simulink model "Sample594"  (R2021b)
settings: Solver=VariableStepAuto  StartTime=0.0  StopTime=10.0  RelTol=1e-3
undefined symbols (not defined in the file): DiscIntNeverNeededParam, magnitude, Newton, Raphson
libraries: simulink x402, pid_lib x98
(part 11 of 14)

== system Sample594/cfblk7/cfblk10/cfblk9/cfblk8 ==
  cfblk1 : Inport
  cfblk6 : Inport  Port=2
  cfblk7 : Inport  Port=3
  cfblk8 : Inport  Port=4
  cfblk3 : simulink/Discrete/Difference  ICPrevInput=0.0  OutMin=[]  OutMax=[]  OutDataTypeStr=Inherit: Inherit via back propagation  OutDataType=fixdt(1, 16)  OutScaling=2^-10  DoSatur=off
  cfblk4 : Sqrt  Operator=rSqrt  AlgorithmType=Newton-Raphson  SaturateOnIntegerOverflow=on
  cfblk5 : Squeeze
  cfblk2 : Outport
  wires:
  cfblk1/1 -> cfblk4/1
  cfblk3/1 -> cfblk2/1
  cfblk6/1 -> cfblk5/1
  cfblk8/1 -> cfblk3/1

== system Sample594/cfblk7/cfblk10/cfblk9/cfblk9 ==
  cfblk1 : Inport
  cfblk11 : Inport  Port=2
  cfblk12 : Inport  Port=3
  cfblk13 : Inport  Port=4
  cfblk14 : Inport  Port=5
  cfblk15 : Inport  Port=6
  cfblk16 : Inport  Port=7
  cfblk10 : simulink/Math Operations/MinMax Running Resettable  Function=min  vinit=0.0
  cfblk18 : Delay  SampleTime=1
  cfblk3 : simulink/Discrete/Tapped Delay  vinit=0.0  samptime=-1  NumDelays=1  DelayOrder=Oldest  includeCurrent=off
  cfblk4 : pid_lib/PID Controller (2DOF)  Controller=PID  Form=Parallel  TimeDomain=Discrete-time  UseExternalTs=off  SampleTime=1  IntegratorMethod=Forward Euler  FilterMethod=Forward Euler  ControllerParametersSource=internal  P=1  I=1  D=0  UseFilter=on  N=100  b=1  c=1  TunerSelectOption=Transfer Function Based (PID Tuner App)  InitialConditionSource=internal  InitialConditionForIntegrator=0  InitialConditionForFilter=0  DifferentiatorICPrevScaledInput=0  ExternalReset=none  TrackingMode=off  Kt=1  LimitOutput=off  SatLimitsSource=internal  UpperSaturationLimit=inf  LowerSaturationLimit=-inf  LinearizeAsGain=off  AntiWindupMode=none  Kb=1  POutMin=[]  POutMax=[]  IOutMin=[]  IOutMax=[]  DOutMin=[]  DOutMax=[]  NOutMin=[]  NOutMax=[]  bOutMin=[]  bOutMax=[]  cOutMin=[]  cOutMax=[]  SumOutMin=[]  SumOutMax=[]  SaturationOutMin=[]  SaturationOutMax=[]  PParamMin=[]  PParamMax=[]  IParamMin=[]  IParamMax=[]  DParamMin=[]  DParamMax=[]  NParamMin=[]  NParamMax=[]  bParamMin=[]  bParamMax=[]  cParamMin=[]  cParamMax=[]  KbParamMin=[]  KbParamMax=[]  KtParamMin=[]  KtParamMax=[]  KbOutMin=[]  KbOutMax=[]  KtOutMin=[]  KtOutMax=[]  IntegratorOutMin=[]  IntegratorOutMax=[]  FilterOutMin=[]  FilterOutMax=[]  SumI1OutMin=[]  SumI1OutMax=[]  SumI2OutMin=[]  SumI2OutMax=[]  SumI3OutMin=[]  SumI3OutMax=[]  SumI4OutMin=[]  SumI4OutMax=[]  SumDOutMin=[]  SumDOutMax=[]  Sum1OutMin=[]  Sum1OutMax=[]  Sum2OutMin=[]  Sum2OutMax=[]  Sum3OutMin=[]  Sum3OutMax=[]  DifferentiatorOutMin=[]  DifferentiatorOutMax=[]  FilterDiffOutCoefMin=[]  FilterDiffOutCoefMax=[]  ReciprocalOutMin=[]  ReciprocalOutMax=[]  SumDenOutMin=[]  SumDenOutMax=[]  SumNumOutMin=[]  SumNumOutMax=[]  DivideOutMin=[]  DivideOutMax=[]  UdiffTsProdOutMin=[]  UdiffTsProdOutMax=[]  NTsProdOutMin=[]  NTsProdOutMax=[]  UintegralTsProdOutMin=[]  UintegralTsProdOutMax=[]  UngainTsProdOutMin=[]  UngainTsProdOutMax=[]  IntegratorContinuousStateAttributes=''  IntegratorStateMustResolveToSignalObject=off  IntegratorRTWStateStorageClass=Auto  FilterContinuousStateAttributes=''  FilterStateMustResolveToSignalObject=off  FilterRTWStateStorageClass=Auto  ParallelPVariant=InternalParameters  IdealPVariant=Disabled  IVariant=InternalParameters  DVariant=InternalParameters  bVariant=InternalParameters  cVariant=InternalParameters  IntegratorVariant=Discrete  SatVariant=Disabled  AWVariant=Passthrough  PCopyVariant=Disabled  TRVariant=Disabled  FdbkBlocksVariant=Forward  IdealPFdbkVariant=Disabled  SatFdbkVariant=Disabled  DerivativeFilterVariant=ForwardEulerFilter  NVariant=InternalParameters  NCopyVariant=Disabled  FilterICVariant=InternalICsFilter  IntegratorICVariant=InternalICs  ExternalResetVariant=Disabled  TRSumVariant=Passthrough  SumFdbkVariant=Disabled  SumVariant=Sum_PID  TsampFilterVariant=InternalTs  TsampNgainVariant=Passthrough  TsampIntegralVariant=Passthrough  ExternalSaturationOutDataTypeStr=Inherit: Same as second input
      settings: SourceProductBaseCode=SL
  cfblk5 : DotProduct  InputSameDT=on  OutDataTypeStr=Inherit: Inherit via internal rule
  cfblk6 : ComplexToMagnitudeAngle
  cfblk7 : Product  Inputs=**
  cfblk8 : Assignment  DiagnosticForDimensions=Warning  IndexOptions=Index vector (dialog)  Indices=1  OutputSizes=1
  cfblk9 : Bias  Bias=[987332324.215911]
  cfblk2 : Outport
  cfblk17 : Outport  Port=2
  wires:
  cfblk3/1 -> cfblk8/1
  cfblk15/1 -> cfblk9/1
  cfblk1/1 -> cfblk4/1
  cfblk12/1 -> cfblk17/1
  cfblk11/1 -> cfblk3/1
  cfblk14/1 -> cfblk6/1
  cfblk9/1 -> cfblk10/1
  cfblk16/1 -> cfblk7/1
  cfblk8/1 -> cfblk10/2
  cfblk5/1 -> cfblk2/1
  cfblk4/1 -> cfblk7/2
  cfblk13/1 -> cfblk5/1
  cfblk7/1 -> cfblk5/2
  cfblk6/1 -> cfblk4/2
  cfblk10/1 -> cfblk18/1
  cfblk18/1 -> cfblk8/2

== system Sample594/cfblk7/cfblk11/cfblk11/cfblk8 ==
  cfblk1 : Inport
  cfblk7 : Inport  Port=2
  cfblk3 : UnaryMinus
  cfblk4 : Sqrt  Operator=rSqrt  AlgorithmType=Newton-Raphson  SaturateOnIntegerOverflow=on
  cfblk5 : Sqrt  Operator=rSqrt  AlgorithmType=Newton-Raphson  SaturateOnIntegerOverflow=on
  cfblk6 : Constant  Value=[773406502.587289]  SampleTime=1
  cfblk2 : Outport
  cfblk8 : Outport  Port=2
  cfblk9 : Outport  Port=3
  wires:
  cfblk6/1 -> cfblk8/1
  cfblk3/1 -> cfblk4/1
  cfblk5/1 -> cfblk2/1
  cfblk1/1 -> cfblk3/1
  cfblk4/1 -> cfblk5/1
  cfblk7/1 -> cfblk9/1

== system Sample594/cfblk7/cfblk11/cfblk9/cfblk8 ==
  cfblk1 : Inport
  cfblk8 : Inport  Port=2
  cfblk9 : Inport  Port=3
  cfblk10 : Delay  SampleTime=1
  cfblk3 : simulink/Discrete/Transfer Fcn Lead or Lag  PoleZ=0.95  ZeroZ=0.75  ICPrevOutput=0.0  ICPrevInput=0.0  DoSatur=off
      settings: SourceProductBaseCode=SL
  cfblk4 : Delay  SampleTime=1
  cfblk5 : Squeeze
  cfblk6 : Sum  Inputs=|++
  cfblk7 : Signum
  cfblk2 : Outport
  wires:
  cfblk6/1 -> cfblk3/1
  cfblk8/1 -> cfblk2/1
  cfblk4/1 -> cfblk7/1
  cfblk3/1 -> cfblk5/1
  cfblk9/1 -> cfblk4/1
  cfblk1/1 -> cfblk6/2
  cfblk5/1 -> cfblk10/1
  cfblk10/1 -> cfblk6/1

== system Sample594/cfblk7/cfblk12/cfblk6/cfblk11 ==
  cfblk1 : Inport
  cfblk10 : Inport  Port=2
  cfblk11 : Inport  Port=3
  cfblk3 : Delay  ShowEnablePort=on  SampleTime=1
      settings: InputPortMap=u0,e6
  cfblk4 : ComplexToMagnitudeAngle
  cfblk5 : Polyval  Coefs=[ +2.081618890e-019, -1.441693666e-014, +4.719686976e-010, -8.536869453e-006, +1.621573104e-001, -8.087801117e+001 ]
  cfblk6 : UnaryMinus
  cfblk7 : Gain  Gain=[975284197.068087]
  cfblk8 : Gain  Gain=[457208272.318980]
  cfblk9 : Constant  Value=[771388824.910894]  SampleTime=1
  cfblk2 : Outport
  cfblk12 : Outport  Port=2
  wires:
  cfblk8/1 -> cfblk3/1
  cfblk9/1 -> cfblk5/1
  cfblk11/1 -> cfblk3/2
  cfblk10/1 -> cfblk8/1
  cfblk4/1 -> cfblk6/1
  cfblk1/1 -> cfblk7/1
  cfblk5/1 -> cfblk12/1
  cfblk6/1 -> cfblk2/1
  cfblk7/1 -> cfblk4/1

== system Sample594/cfblk7/cfblk12/cfblk6/cfblk12 ==
  cfblk1 : Inport
  cfblk11 : Inport  Port=2
  cfblk12 : Inport  Port=3
  cfblk13 : Inport  Port=4
  cfblk14 : Inport  Port=5
  cfblk15 : Inport  Port=6
  cfblk10 : Constant  Value=[-798573774.172849]  SampleTime=1
  cfblk3 : simulink/Discrete/Difference  ICPrevInput=0.0  OutMin=[]  OutMax=[]  OutDataTypeStr=Inherit: Inherit via back propagation  OutDataType=fixdt(1, 16)  OutScaling=2^-10  DoSatur=off
  cfblk4 : simulink/Math Operations/Slider Gain  gain=1  low=0  high=2
  cfblk5 : PermuteDimensions
  cfblk6 : Rounding
  cfblk7 : ComplexToMagnitudeAngle
  cfblk8 : Product  Inputs=*
  cfblk9 : Constant  Value=[339268428.821367]  SampleTime=1
  cfblk2 : Outport
  cfblk16 : Outport  Port=2
  cfblk17 : Outport  Port=3
  wires:
  cfblk12/1 -> cfblk3/1
  cfblk10/1 -> cfblk2/1
  cfblk15/1 -> cfblk6/1
  cfblk7/1 -> cfblk16/1
  cfblk8/1 -> cfblk4/1
  cfblk4/1 -> cfblk17/1
  cfblk11/1 -> cfblk8/1
  cfblk5/1 -> cfblk7/1
  cfblk14/1 -> cfblk5/1

== system Sample594/cfblk7/cfblk12/cfblk6/cfblk13 ==
  cfblk1 : Inport
  cfblk14 : Inport  Port=2
  cfblk10 : Sum  Inputs=+
  cfblk11 : Trigonometry
  cfblk12 : Constant  Value=[-924732541.629260]  SampleTime=1
  cfblk13 : Constant  Value=[218240714.149270]  SampleTime=1
  cfblk15 : Delay  SampleTime=1
  cfblk3 : DiscreteTransferFcn  SampleTime=1
  cfblk4 : pid_lib/PID Controller (2DOF)  Controller=PID  Form=Parallel  TimeDomain=Discrete-time  UseExternalTs=off  SampleTime=1  IntegratorMethod=Forward Euler  FilterMethod=Forward Euler  ControllerParametersSource=internal  P=1  I=1  D=0  UseFilter=on  N=100  b=1  c=1  TunerSelectOption=Transfer Function Based (PID Tuner App)  InitialConditionSource=internal  InitialConditionForIntegrator=0  InitialConditionForFilter=0  DifferentiatorICPrevScaledInput=0  ExternalReset=none  TrackingMode=off  Kt=1  LimitOutput=off  SatLimitsSource=internal  UpperSaturationLimit=inf  LowerSaturationLimit=-inf  LinearizeAsGain=off  AntiWindupMode=none  Kb=1  POutMin=[]  POutMax=[]  IOutMin=[]  IOutMax=[]  DOutMin=[]  DOutMax=[]  NOutMin=[]  NOutMax=[]  bOutMin=[]  bOutMax=[]  cOutMin=[]  cOutMax=[]  SumOutMin=[]  SumOutMax=[]  SaturationOutMin=[]  SaturationOutMax=[]  PParamMin=[]  PParamMax=[]  IParamMin=[]  IParamMax=[]  DParamMin=[]  DParamMax=[]  NParamMin=[]  NParamMax=[]  bParamMin=[]  bParamMax=[]  cParamMin=[]  cParamMax=[]  KbParamMin=[]  KbParamMax=[]  KtParamMin=[]  KtParamMax=[]  KbOutMin=[]  KbOutMax=[]  KtOutMin=[]  KtOutMax=[]  IntegratorOutMin=[]  IntegratorOutMax=[]  FilterOutMin=[]  FilterOutMax=[]  SumI1OutMin=[]  SumI1OutMax=[]  SumI2OutMin=[]  SumI2OutMax=[]  SumI3OutMin=[]  SumI3OutMax=[]  SumI4OutMin=[]  SumI4OutMax=[]  SumDOutMin=[]  SumDOutMax=[]  Sum1OutMin=[]  Sum1OutMax=[]  Sum2OutMin=[]  Sum2OutMax=[]  Sum3OutMin=[]  Sum3OutMax=[]  DifferentiatorOutMin=[]  DifferentiatorOutMax=[]  FilterDiffOutCoefMin=[]  FilterDiffOutCoefMax=[]  ReciprocalOutMin=[]  ReciprocalOutMax=[]  SumDenOutMin=[]  SumDenOutMax=[]  SumNumOutMin=[]  SumNumOutMax=[]  DivideOutMin=[]  DivideOutMax=[]  UdiffTsProdOutMin=[]  UdiffTsProdOutMax=[]  NTsProdOutMin=[]  NTsProdOutMax=[]  UintegralTsProdOutMin=[]  UintegralTsProdOutMax=[]  UngainTsProdOutMin=[]  UngainTsProdOutMax=[]  IntegratorContinuousStateAttributes=''  IntegratorStateMustResolveToSignalObject=off  IntegratorRTWStateStorageClass=Auto  FilterContinuousStateAttributes=''  FilterStateMustResolveToSignalObject=off  FilterRTWStateStorageClass=Auto  ParallelPVariant=InternalParameters  IdealPVariant=Disabled  IVariant=InternalParameters  DVariant=InternalParameters  bVariant=InternalParameters  cVariant=InternalParameters  IntegratorVariant=Discrete  SatVariant=Disabled  AWVariant=Passthrough  PCopyVariant=Disabled  TRVariant=Disabled  FdbkBlocksVariant=Forward  IdealPFdbkVariant=Disabled  SatFdbkVariant=Disabled  DerivativeFilterVariant=ForwardEulerFilter  NVariant=InternalParameters  NCopyVariant=Disabled  FilterICVariant=InternalICsFilter  IntegratorICVariant=InternalICs  ExternalResetVariant=Disabled  TRSumVariant=Passthrough  SumFdbkVariant=Disabled  SumVariant=Sum_PID  TsampFilterVariant=InternalTs  TsampNgainVariant=Passthrough  TsampIntegralVariant=Passthrough  ExternalSaturationOutDataTypeStr=Inherit: Same as second input
      settings: SourceProductBaseCode=SL
  cfblk5 : DiscreteIntegrator  ICPrevOutput=DiscIntNeverNeededParam  ICPrevScaledInput=DiscIntNeverNeededParam
  cfblk6 : simulink/Discrete/Transfer Fcn First Order  PoleZ=0.95  ICPrevOutput=0.0  DoSatur=off
  cfblk7 : simulink/Discrete/Transfer Fcn First Order  PoleZ=0.95  ICPrevOutput=0.0  DoSatur=off
  cfblk8 : Bias  Bias=[-119324270.093714]
  cfblk9 : Math  Operator=hypot  SaturateOnIntegerOverflow=on
  cfblk2 : Outport
  wires:
  cfblk6/1 -> cfblk11/1
  cfblk11/1 -> cfblk5/1
  cfblk12/1 -> cfblk9/1
  cfblk5/1 -> cfblk4/1
  cfblk1/1 -> cfblk6/1
  cfblk10/1 -> cfblk2/1
  cfblk4/1 -> cfblk3/1
  cfblk13/1 -> cfblk4/2
  cfblk14/1 -> cfblk8/1
  cfblk8/1 -> cfblk10/1
  cfblk7/1 -> cfblk9/2
  cfblk9/1 -> cfblk15/1
  cfblk15/1 -> cfblk7/1

== system Sample594/cfblk7/cfblk12/cfblk7/cfblk12 ==
  cfblk1 : Inport
  cfblk9 : Inport  Port=2
  cfblk10 : Inport  Port=3
  cfblk11 : Delay  SampleTime=1
  cfblk3 : pid_lib/PID Controller  Controller=PID  Form=Parallel  TimeDomain=Discrete-time  UseExternalTs=off  SampleTime=1  IntegratorMethod=Forward Euler  FilterMethod=Forward Euler  ControllerParametersSource=internal  P=1  I=1  D=0  UseFilter=on  N=100  TunerSelectOption=Transfer Function Based (PID Tuner App)  InitialConditionSource=internal  InitialConditionForIntegrator=0  InitialConditionForFilter=0  DifferentiatorICPrevScaledInput=0  ExternalReset=none  TrackingMode=off  Kt=1  LimitOutput=off  SatLimitsSource=internal  UpperSaturationLimit=inf  LowerSaturationLimit=-inf  LinearizeAsGain=off  AntiWindupMode=none  Kb=1  POutMin=[]  POutMax=[]  IOutMin=[]  IOutMax=[]  DOutMin=[]  DOutMax=[]  NOutMin=[]  NOutMax=[]  SumOutMin=[]  SumOutMax=[]  SaturationOutMin=[]  SaturationOutMax=[]  PParamMin=[]  PParamMax=[]  IParamMin=[]  IParamMax=[]  DParamMin=[]  DParamMax=[]  NParamMin=[]  NParamMax=[]  KbParamMin=[]  KbParamMax=[]  KtParamMin=[]  KtParamMax=[]  KbOutMin=[]  KbOutMax=[]  KtOutMin=[]  KtOutMax=[]  IntegratorOutMin=[]  IntegratorOutMax=[]  FilterOutMin=[]  FilterOutMax=[]  SumI1OutMin=[]  SumI1OutMax=[]  SumI2OutMin=[]  SumI2OutMax=[]  SumI3OutMin=[]  SumI3OutMax=[]  SumI4OutMin=[]  SumI4OutMax=[]  SumDOutMin=[]  SumDOutMax=[]  DifferentiatorOutMin=[]  DifferentiatorOutMax=[]  FilterDiffOutCoefMin=[]  FilterDiffOutCoefMax=[]  ReciprocalOutMin=[]  ReciprocalOutMax=[]  SumDenOutMin=[]  SumDenOutMax=[]  SumNumOutMin=[]  SumNumOutMax=[]  DivideOutMin=[]  DivideOutMax=[]  UdiffTsProdOutMin=[]  UdiffTsProdOutMax=[]  NTsProdOutMin=[]  NTsProdOutMax=[]  UintegralTsProdOutMin=[]  UintegralTsProdOutMax=[]  UngainTsProdOutMin=[]  UngainTsProdOutMax=[]  IntegratorContinuousStateAttributes=''  IntegratorStateMustResolveToSignalObject=off  IntegratorRTWStateStorageClass=Auto  FilterContinuousStateAttributes=''  FilterStateMustResolveToSignalObject=off  FilterRTWStateStorageClass=Auto  ParallelPVariant=InternalParameters  IdealPVariant=Disabled  IVariant=InternalParameters  DVariant=InternalParameters  IntegratorVariant=Discrete  SatVariant=Disabled  AWVariant=Passthrough  PCopyVariant=Disabled  TRVariant=Disabled  FdbkBlocksVariant=Forward  IdealPFdbkVariant=Disabled  SatFdbkVariant=Disabled  DerivativeFilterVariant=ForwardEulerFilter  NVariant=InternalParameters  NCopyVariant=Disabled  FilterICVariant=InternalICsFilter  IntegratorICVariant=InternalICs  ExternalResetVariant=Disabled  TRSumVariant=Passthrough  SumFdbkVariant=Disabled  SumVariant=Sum_PID  TsampFilterVariant=InternalTs  TsampNgainVariant=Passthrough  TsampIntegralVariant=Passthrough  ExternalSaturationOutDataTypeStr=Inherit: Same as second input
  cfblk4 : Rounding
  cfblk5 : ComplexToRealImag
  cfblk6 : Sqrt  SaturateOnIntegerOverflow=on
  cfblk7 : Product  Inputs=**
  cfblk8 : Reshape
  cfblk2 : Outport
  wires:
  cfblk1/1 -> cfblk8/1
  cfblk3/1 -> cfblk7/1
  cfblk10/1 -> cfblk6/1
  cfblk9/1 -> cfblk4/1
  cfblk4/1 -> cfblk5/1
  cfblk6/1 -> cfblk7/2
  cfblk5/1 -> cfblk2/1
  cfblk7/1 -> cfblk11/1
  cfblk11/1 -> cfblk3/1

== system Sample594/cfblk7/cfblk12/cfblk7/cfblk13 ==
  cfblk1 : Inport
  cfblk13 : Inport  Port=2
  cfblk14 : Inport  Port=3
  cfblk15 : Inport  Port=4
  cfblk10 : ComplexToRealImag
  cfblk11 : Signum
  cfblk12 : simulink/Math Operations/Slider Gain  gain=1  low=0  high=2
  cfblk16 : Delay  SampleTime=1
  cfblk17 : Delay  SampleTime=1
  cfblk18 : Delay  SampleTime=1
  cfblk3 : DiscreteFir  SampleTime=1
  cfblk4 : simulink/Discrete/Transfer Fcn Real Zero  ZeroZ=0.75  ICPrevInput=0.0  DoSatur=off
      settings: SourceProductBaseCode=SL
  cfblk5 : DiscreteTransferFcn  SampleTime=1
  cfblk6 : simulink/Discrete/Difference  ICPrevInput=0.0  OutMin=[]  OutMax=[]  OutDataTypeStr=Inherit: Inherit via back propagation  OutDataType=fixdt(1, 16)  OutScaling=2^-10  DoSatur=off
  cfblk7 : pid_lib/PID Controller  Controller=PID  Form=Parallel  TimeDomain=Discrete-time  UseExternalTs=off  SampleTime=1  IntegratorMethod=Forward Euler  FilterMethod=Forward Euler  ControllerParametersSource=internal  P=1  I=1  D=0  UseFilter=on  N=100  TunerSelectOption=Transfer Function Based (PID Tuner App)  InitialConditionSource=internal  InitialConditionForIntegrator=0  InitialConditionForFilter=0  DifferentiatorICPrevScaledInput=0  ExternalReset=none  TrackingMode=off  Kt=1  LimitOutput=off  SatLimitsSource=internal  UpperSaturationLimit=inf  LowerSaturationLimit=-inf  LinearizeAsGain=off  AntiWindupMode=none  Kb=1  POutMin=[]  POutMax=[]  IOutMin=[]  IOutMax=[]  DOutMin=[]  DOutMax=[]  NOutMin=[]  NOutMax=[]  SumOutMin=[]  SumOutMax=[]  SaturationOutMin=[]  SaturationOutMax=[]  PParamMin=[]  PParamMax=[]  IParamMin=[]  IParamMax=[]  DParamMin=[]  DParamMax=[]  NParamMin=[]  NParamMax=[]  KbParamMin=[]  KbParamMax=[]  KtParamMin=[]  KtParamMax=[]  KbOutMin=[]  KbOutMax=[]  KtOutMin=[]  KtOutMax=[]  IntegratorOutMin=[]  IntegratorOutMax=[]  FilterOutMin=[]  FilterOutMax=[]  SumI1OutMin=[]  SumI1OutMax=[]  SumI2OutMin=[]  SumI2OutMax=[]  SumI3OutMin=[]  SumI3OutMax=[]  SumI4OutMin=[]  SumI4OutMax=[]  SumDOutMin=[]  SumDOutMax=[]  DifferentiatorOutMin=[]  DifferentiatorOutMax=[]  FilterDiffOutCoefMin=[]  FilterDiffOutCoefMax=[]  ReciprocalOutMin=[]  ReciprocalOutMax=[]  SumDenOutMin=[]  SumDenOutMax=[]  SumNumOutMin=[]  SumNumOutMax=[]  DivideOutMin=[]  DivideOutMax=[]  UdiffTsProdOutMin=[]  UdiffTsProdOutMax=[]  NTsProdOutMin=[]  NTsProdOutMax=[]  UintegralTsProdOutMin=[]  UintegralTsProdOutMax=[]  UngainTsProdOutMin=[]  UngainTsProdOutMax=[]  IntegratorContinuousStateAttributes=''  IntegratorStateMustResolveToSignalObject=off  IntegratorRTWStateStorageClass=Auto  FilterContinuousStateAttributes=''  FilterStateMustResolveToSignalObject=off  FilterRTWStateStorageClass=Auto  ParallelPVariant=InternalParameters  IdealPVariant=Disabled  IVariant=InternalParameters  DVariant=InternalParameters  IntegratorVariant=Discrete  SatVariant=Disabled  AWVariant=Passthrough  PCopyVariant=Disabled  TRVariant=Disabled  FdbkBlocksVariant=Forward  IdealPFdbkVariant=Disabled  SatFdbkVariant=Disabled  DerivativeFilterVariant=ForwardEulerFilter  NVariant=InternalParameters  NCopyVariant=Disabled  FilterICVariant=InternalICsFilter  IntegratorICVariant=InternalICs  ExternalResetVariant=Disabled  TRSumVariant=Passthrough  SumFdbkVariant=Disabled  SumVariant=Sum_PID  TsampFilterVariant=InternalTs  TsampNgainVariant=Passthrough  TsampIntegralVariant=Passthrough  ExternalSaturationOutDataTypeStr=Inherit: Same as second input
  cfblk8 : simulink/Discrete/Transfer Fcn Lead or Lag  PoleZ=0.95  ZeroZ=0.75  ICPrevOutput=0.0  ICPrevInput=0.0  DoSatur=off
      settings: SourceProductBaseCode=SL
  cfblk9 : DotProduct  InputSameDT=on  OutDataTypeStr=Inherit: Inherit via internal rule
  cfblk2 : Outport
  wires:
  cfblk11/1 -> cfblk3/1
  cfblk7/1 -> cfblk12/1
  cfblk15/1 -> cfblk4/1
  cfblk4/1 -> cfblk10/1
  cfblk1/1 -> cfblk9/1
  cfblk14/1 -> cfblk2/1
  cfblk8/1 -> cfblk6/1
  cfblk9/1 -> cfblk11/1
  cfblk5/1 -> cfblk8/1
  cfblk3/1 -> cfblk16/1
  cfblk16/1 -> cfblk9/2
  cfblk6/1 -> cfblk17/1
  cfblk17/1 -> cfblk5/1
  cfblk12/1 -> cfblk18/1
  cfblk18/1 -> cfblk7/1

== system Sample594/cfblk7/cfblk12/cfblk7/cfblk14 ==
  cfblk1 : Inport
  cfblk6 : Inport  Port=2
  cfblk7 : Inport  Port=3
  cfblk8 : Inport  Port=4
  cfblk3 : simulink/Discrete/Transfer Fcn Real Zero  ZeroZ=0.75  ICPrevInput=0.0  DoSatur=off
      settings: SourceProductBaseCode=SL
  cfblk4 : Sum  Inputs=|++
  cfblk5 : Sum  Inputs=+
  cfblk2 : Outport
  cfblk9 : Outport  Port=2
  wires:
  cfblk7/1 -> cfblk9/1
  cfblk1/1 -> cfblk4/1
  cfblk5/1 -> cfblk2/1
  cfblk8/1 -> cfblk4/2
  cfblk3/1 -> cfblk5/1
  cfblk4/1 -> cfblk3/1

== system Sample594/cfblk7/cfblk12/cfblk8/cfblk10 ==
  cfblk1 : Inport
  Action Port : ActionPort  ActionPortLabel=else
  cfblk11 : Delay
  cfblk12 : Delay
  cfblk3 : simulink/Discrete/Tapped Delay  vinit=0.0  samptime=-1  NumDelays=1  DelayOrder=Oldest  includeCurrent=off
  cfblk4 : Math  Operator=pow  SaturateOnIntegerOverflow=on
  cfblk5 : Assignment  DiagnosticForDimensions=Warning  IndexOptions=Index vector (dialog)  Indices=1  OutputSizes=1
  cfblk6 : Product
  cfblk7 : Bias  Bias=[-175070378.275236]
  cfblk8 : Sin  TimeSource=Use external signal  SampleTime=0
  cfblk9 : Constant  Value=[-888949273.782798]  SampleTime=1
  cfblk2 : Outport
  cfblk10 : Outport  Port=2
  wires:
  cfblk7/1 -> cfblk2/1
  cfblk8/1 -> cfblk7/1, cfblk11/1
  cfblk5/1 -> cfblk3/1
  cfblk6/1 -> cfblk5/1
  cfblk4/1 -> cfblk8/1
  cfblk9/1 -> cfblk10/1, cfblk4/2
  cfblk3/1 -> cfblk4/1, cfblk12/1
  cfblk1/1 -> cfblk6/1
  cfblk11/1 -> cfblk5/2
  cfblk12/1 -> cfblk6/2

== system Sample594/cfblk7/cfblk12/cfblk8/cfblk6 ==
  cfblk1 : Inport
  cfblk3 : Product  Inputs=**
  cfblk4 : Abs
  cfblk5 : Sin  TimeSource=Use external signal  SampleTime=0
  cfblk6 : Signum
  cfblk7 : Constant  Value=[45329702.719841]  SampleTime=1
  cfblk2 : Outport
  wires:
  cfblk7/1 -> cfblk6/1
  cfblk5/1 -> cfblk3/1
  cfblk6/1 -> cfblk3/2
  cfblk1/1 -> cfblk5/1
  cfblk3/1 -> cfblk2/1, cfblk4/1

== system Sample594/cfblk7/cfblk12/cfblk8/cfblk9 ==
  cfblk1 : Inport
  cfblk6 : Inport  Port=2
  cfblk7 : Inport  Port=3
  cfblk8 : Inport  Port=4
  Action Port : ActionPort  ActionPortLabel=if(u1 >= 0)
  cfblk3 : simulink/Discrete/Transfer Fcn Lead or Lag  PoleZ=0.95  ZeroZ=0.75  ICPrevOutput=0.0  ICPrevInput=0.0  DoSatur=off
      settings: SourceProductBaseCode=SL
  cfblk4 : ComplexToMagnitudeAngle
  cfblk5 : Constant  Value=[-986884482.511497]  SampleTime=1
  cfblk2 : Outport
  cfblk9 : Outport  Port=2
  cfblk10 : Outport  Port=3
  cfblk11 : Outport  Port=4
  wires:
  cfblk8/1 -> cfblk2/1
  cfblk4/1 -> cfblk3/1
  cfblk1/1 -> cfblk4/1
  cfblk7/1 -> cfblk11/1
  cfblk3/1 -> cfblk10/1
  cfblk6/1 -> cfblk9/1

== system Sample594/cfblk7/cfblk12/cfblk9/cfblk9 ==
  cfblk1 : Inport
  cfblk12 : Inport  Port=2
  cfblk10 : Constant  Value=[695376097.149891]  SampleTime=1
  cfblk11 : Constant  Value=[626013830.058781]  SampleTime=1
  cfblk14 : Delay  SampleTime=1
  cfblk15 : Delay  SampleTime=1
  cfblk3 : DiscreteStateSpace
  cfblk4 : Sum  Inputs=|++
  cfblk5 : MinMax  Function=max
  cfblk6 : Product  Inputs=**
  cfblk7 : Sqrt  SaturateOnIntegerOverflow=on
  cfblk8 : Sqrt  SaturateOnIntegerOverflow=on
  cfblk9 : Product  Inputs=*
  cfblk2 : Outport
  cfblk13 : Outport  Port=2
  wires:
  cfblk7/1 -> cfblk4/1
  cfblk6/1 -> cfblk13/1
  cfblk4/1 -> cfblk5/1
  cfblk8/1 -> cfblk2/1
  cfblk10/1 -> cfblk6/1
  cfblk12/1 -> cfblk6/2
  cfblk11/1 -> cfblk7/1
  cfblk3/1 -> cfblk9/1
  cfblk1/1 -> cfblk8/1
  cfblk9/1 -> cfblk14/1
  cfblk14/1 -> cfblk3/1
  cfblk5/1 -> cfblk15/1
  cfblk15/1 -> cfblk4/2

== system Sample594/cfblk7/cfblk13/cfblk11/cfblk10 ==
  cfblk1 : Inport
  cfblk13 : Inport  Port=2
  cfblk14 : Inport  Port=3
  cfblk15 : Inport  Port=4
  cfblk10 : Product  Inputs=**
  cfblk11 : Polyval  Coefs=[ +2.081618890e-019, -1.441693666e-014, +4.719686976e-010, -8.536869453e-006, +1.621573104e-001, -8.087801117e+001 ]
  cfblk12 : Constant  Value=[481756788.873973]  SampleTime=1
  cfblk16 : Delay  SampleTime=1
  cfblk3 : Delay  DelayLengthSource=Input port  SampleTime=1
      settings: InputPortMap=u0,p1
  cfblk4 : DiscreteFilter  SampleTime=1
  cfblk5 : DiscreteZeroPole  Poles=[0 0.5]  Gain=1
  cfblk6 : UnitDelay  HasFrameUpgradeWarning=on
  cfblk7 : Assignment  DiagnosticForDimensions=Warning  IndexOptions=Index vector (dialog)  Indices=1  OutputSizes=1
  cfblk8 : Sum  Inputs=|++
  cfblk9 : Product
  cfblk2 : Outport
  wires:
  cfblk11/1 -> cfblk10/1
  cfblk12/1 -> cfblk6/1
  cfblk7/1 -> cfblk4/1
  cfblk8/1 -> cfblk7/1
  cfblk15/1 -> cfblk2/1
  cfblk14/1 -> cfblk3/1
  cfblk5/1 -> cfblk3/2
  cfblk10/1 -> cfblk7/2
  cfblk13/1 -> cfblk5/1
  cfblk1/1 -> cfblk11/1
  cfblk9/1 -> cfblk8/1
  cfblk6/1 -> cfblk9/1
  cfblk3/1 -> cfblk9/2, cfblk8/2
  cfblk4/1 -> cfblk16/1
  cfblk16/1 -> cfblk10/2

== system Sample594/cfblk7/cfblk13/cfblk11/cfblk11 ==
  cfblk1 : Inport
  cfblk7 : Inport  Port=2
  cfblk3 : DiscreteFir  SampleTime=1
  cfblk4 : Polyval  Coefs=[ +2.081618890e-019, -1.441693666e-014, +4.719686976e-010, -8.536869453e-006, +1.621573104e-001, -8.087801117e+001 ]
  cfblk5 : Math  Operator=transpose  SaturateOnIntegerOverflow=on
  cfblk6 : Constant  Value=[-39723787.127016]  SampleTime=1
  cfblk2 : Outport
  wires:
  cfblk4/1 -> cfblk2/1
  cfblk1/1 -> cfblk3/1
  cfblk6/1 -> cfblk4/1
  cfblk3/1 -> cfblk5/1

== system Sample594/cfblk7/cfblk13/cfblk11/cfblk12 ==
  cfblk1 : Inport
  cfblk12 : Inport  Port=2
  cfblk13 : Inport  Port=3
  cfblk14 : Inport  Port=4
  cfblk10 : MinMax  Function=max  Inputs=2
  cfblk11 : Sum
  cfblk{3,6,15..17} (5 alike) : Delay  SampleTime=1
  cfblk4 : simulink/Discrete/Transfer Fcn Lead or Lag  PoleZ=0.95  ZeroZ=0.75  ICPrevOutput=0.0  ICPrevInput=0.0  DoSatur=off
      settings: SourceProductBaseCode=SL
  cfblk5 : Delay  ShowEnablePort=on  SampleTime=1
      settings: InputPortMap=u0,e6
  cfblk7 : DiscreteIntegrator  ICPrevOutput=DiscIntNeverNeededParam  ICPrevScaledInput=DiscIntNeverNeededParam
  cfblk8 : simulink/Discrete/Transfer Fcn First Order  PoleZ=0.95  ICPrevOutput=0.0  DoSatur=off
  cfblk9 : Sum  Inputs=--
  cfblk2 : Outport
  wires:
  cfblk10/1 -> cfblk8/1
  cfblk6/1 -> cfblk7/1
  cfblk1/1 -> cfblk2/1
  cfblk3/1 -> cfblk10/1
  cfblk7/1 -> cfblk11/1, cfblk9/2
  cfblk13/1 -> cfblk3/1
  cfblk5/1 -> cfblk9/1
  cfblk14/1 -> cfblk11/2
  cfblk12/1 -> cfblk5/1
  cfblk4/1 -> cfblk5/2
  cfblk8/1 -> cfblk15/1
  cfblk15/1 -> cfblk10/2
  cfblk9/1 -> cfblk16/1
  cfblk16/1 -> cfblk4/1
  cfblk11/1 -> cfblk17/1
  cfblk17/1 -> cfblk6/1

== system Sample594/cfblk7/cfblk13/cfblk11/cfblk13 ==
  cfblk1 : Inport
  cfblk12 : Inport  Port=2
  cfblk13 : Inport  Port=3
  cfblk14 : Inport  Port=4
  cfblk15 : Inport  Port=5
  cfblk16 : Inport  Port=6
  cfblk10 : Polyval  Coefs=[ +2.081618890e-019, -1.441693666e-014, +4.719686976e-010, -8.536869453e-006, +1.621573104e-001, -8.087801117e+001 ]
  cfblk11 : Constant  Value=[352412146.221429]  SampleTime=1
  cfblk3 : Delay  DelayLengthSource=Input port  SampleTime=1
      settings: InputPortMap=u0,p1
  cfblk4 : DiscreteTransferFcn  SampleTime=1
  cfblk5 : DiscreteFilter  SampleTime=1
  cfblk6 : UnitDelay  HasFrameUpgradeWarning=on
  cfblk7 : DiscreteStateSpace
  cfblk8 : MinMax  Function=max  Inputs=3
  cfblk9 : Trigonometry
  cfblk2 : Outport
  cfblk17 : Outport  Port=2
  wires:
  cfblk10/1 -> cfblk17/1
  cfblk12/1 -> cfblk4/1
  cfblk11/1 -> cfblk6/1
  cfblk1/1 -> cfblk5/1
  cfblk3/1 -> cfblk2/1
  cfblk9/1 -> cfblk8/1
  cfblk6/1 -> cfblk8/2
  cfblk15/1 -> cfblk9/1
  cfblk14/1 -> cfblk10/1
  cfblk13/1 -> cfblk3/1
  cfblk16/1 -> cfblk7/1
  cfblk4/1 -> cfblk3/2
  cfblk7/1 -> cfblk8/3

== system Sample594/cfblk7/cfblk13/cfblk11/cfblk15 ==
  cfblk1 : Inport
  Action Port : ActionPort  ActionPortLabel=if(u1 >= 0)
  cfblk3 : Polyval  Coefs=[ +2.081618890e-019, -1.441693666e-014, +4.719686976e-010, -8.536869453e-006, +1.621573104e-001, -8.087801117e+001 ]
  cfblk4 : Squeeze
  cfblk5 : Constant  Value=[102347912.786067]  SampleTime=1
  cfblk2 : Outport
  cfblk6 : Outport  Port=2
  cfblk7 : Outport  Port=3
  wires:
  cfblk1/1 -> cfblk3/1, cfblk2/1
  cfblk3/1 -> cfblk6/1
  cfblk5/1 -> cfblk4/1
  cfblk4/1 -> cfblk7/1

== system Sample594/cfblk7/cfblk13/cfblk11/cfblk16 ==
  cfblk1 : Inport
  cfblk10 : Inport  Port=2
  cfblk11 : Inport  Port=3
  cfblk12 : Inport  Port=4
  Action Port : ActionPort  ActionPortLabel=else
  cfblk3 : DiscreteZeroPole  Poles=[0 0.5]  Gain=1  SampleTime=-1
  cfblk4 : pid_lib/PID Controller (2DOF)  Controller=PID  Form=Parallel  TimeDomain=Discrete-time  UseExternalTs=off  SampleTime=-1  IntegratorMethod=Forward Euler  FilterMethod=Forward Euler  ControllerParametersSource=internal  P=1  I=1  D=0  UseFilter=on  N=100  b=1  c=1  TunerSelectOption=Transfer Function Based (PID Tuner App)  InitialConditionSource=internal  InitialConditionForIntegrator=0  InitialConditionForFilter=0  DifferentiatorICPrevScaledInput=0  ExternalReset=none  TrackingMode=off  Kt=1  LimitOutput=off  SatLimitsSource=internal  UpperSaturationLimit=inf  LowerSaturationLimit=-inf  LinearizeAsGain=off  AntiWindupMode=none  Kb=1  POutMin=[]  POutMax=[]  IOutMin=[]  IOutMax=[]  DOutMin=[]  DOutMax=[]  NOutMin=[]  NOutMax=[]  bOutMin=[]  bOutMax=[]  cOutMin=[]  cOutMax=[]  SumOutMin=[]  SumOutMax=[]  SaturationOutMin=[]  SaturationOutMax=[]  PParamMin=[]  PParamMax=[]  IParamMin=[]  IParamMax=[]  DParamMin=[]  DParamMax=[]  NParamMin=[]  NParamMax=[]  bParamMin=[]  bParamMax=[]  cParamMin=[]  cParamMax=[]  KbParamMin=[]  KbParamMax=[]  KtParamMin=[]  KtParamMax=[]  KbOutMin=[]  KbOutMax=[]  KtOutMin=[]  KtOutMax=[]  IntegratorOutMin=[]  IntegratorOutMax=[]  FilterOutMin=[]  FilterOutMax=[]  SumI1OutMin=[]  SumI1OutMax=[]  SumI2OutMin=[]  SumI2OutMax=[]  SumI3OutMin=[]  SumI3OutMax=[]  SumI4OutMin=[]  SumI4OutMax=[]  SumDOutMin=[]  SumDOutMax=[]  Sum1OutMin=[]  Sum1OutMax=[]  Sum2OutMin=[]  Sum2OutMax=[]  Sum3OutMin=[]  Sum3OutMax=[]  DifferentiatorOutMin=[]  DifferentiatorOutMax=[]  FilterDiffOutCoefMin=[]  FilterDiffOutCoefMax=[]  ReciprocalOutMin=[]  ReciprocalOutMax=[]  SumDenOutMin=[]  SumDenOutMax=[]  SumNumOutMin=[]  SumNumOutMax=[]  DivideOutMin=[]  DivideOutMax=[]  UdiffTsProdOutMin=[]  UdiffTsProdOutMax=[]  NTsProdOutMin=[]  NTsProdOutMax=[]  UintegralTsProdOutMin=[]  UintegralTsProdOutMax=[]  UngainTsProdOutMin=[]  UngainTsProdOutMax=[]  IntegratorContinuousStateAttributes=''  IntegratorStateMustResolveToSignalObject=off  IntegratorRTWStateStorageClass=Auto  FilterContinuousStateAttributes=''  FilterStateMustResolveToSignalObject=off  FilterRTWStateStorageClass=Auto  ParallelPVariant=InternalParameters  IdealPVariant=Disabled  IVariant=InternalParameters  DVariant=InternalParameters  bVariant=InternalParameters  cVariant=InternalParameters  IntegratorVariant=Discrete  SatVariant=Disabled  AWVariant=Passthrough  PCopyVariant=Disabled  TRVariant=Disabled  FdbkBlocksVariant=Forward  IdealPFdbkVariant=Disabled  SatFdbkVariant=Disabled  DerivativeFilterVariant=ForwardEulerFilter  NVariant=InternalParameters  NCopyVariant=Disabled  FilterICVariant=InternalICsFilter  IntegratorICVariant=InternalICs  ExternalResetVariant=Disabled  TRSumVariant=Passthrough  SumFdbkVariant=Disabled  SumVariant=Sum_PID  TsampFilterVariant=InternalTs  TsampNgainVariant=Passthrough  TsampIntegralVariant=Passthrough  ExternalSaturationOutDataTypeStr=Inherit: Same as second input
      settings: SourceProductBaseCode=SL
  cfblk5 : DiscreteStateSpace  SampleTime=-1
  cfblk6 : Sum
  cfblk7 : Abs
  cfblk8 : Sin  TimeSource=Use external signal  SampleTime=0
  cfblk9 : Constant  Value=[-545086462.120134]  SampleTime=1
  cfblk2 : Outport
  wires:
  cfblk4/1 -> cfblk2/1
  cfblk8/1 -> cfblk7/1
  cfblk11/1 -> cfblk4/1
  cfblk3/1 -> cfblk6/1
  cfblk12/1 -> cfblk3/1
  cfblk10/1 -> cfblk4/2
  cfblk9/1 -> cfblk6/2
  cfblk1/1 -> cfblk8/1
  cfblk7/1 -> cfblk5/1

== system Sample594/cfblk7/cfblk13/cfblk12/cfblk10 ==
  cfblk1 : Inport
  cfblk8 : Inport  Port=2
  cfblk3 : Delay  DelayLengthSource=Input port  SampleTime=1
      settings: InputPortMap=u0,p1
  cfblk4 : simulink/Math Operations/MinMax Running Resettable  Function=min  vinit=0.0
  cfblk5 : MinMax
  cfblk6 : UnaryMinus
  cfblk7 : Sqrt  Operator=rSqrt  AlgorithmType=Newton-Raphson  SaturateOnIntegerOverflow=on
  cfblk9 : Delay  SampleTime=1
  cfblk2 : Outport
  wires:
  cfblk1/1 -> cfblk6/1
  cfblk8/1 -> cfblk5/1
  cfblk4/1 -> cfblk7/1
  cfblk6/1 -> cfblk3/1, cfblk4/2
  cfblk3/1 -> cfblk4/1
  cfblk5/1 -> cfblk2/1
  cfblk7/1 -> cfblk9/1
  cfblk9/1 -> cfblk3/2

== system Sample594/cfblk7/cfblk13/cfblk12/cfblk11 ==
  cfblk1 : Inport
  cfblk10 : Inport  Port=2
  cfblk11 : Inport  Port=3
  cfblk12 : Delay  SampleTime=1
  cfblk3 : simulink/Discrete/Difference  ICPrevInput=0.0  OutMin=[]  OutMax=[]  OutDataTypeStr=Inherit: Inherit via back propagation  OutDataType=fixdt(1, 16)  OutScaling=2^-10  DoSatur=off
  cfblk4 : simulink/Discrete/Transfer Fcn First Order  PoleZ=0.95  ICPrevOutput=0.0  DoSatur=off
  cfblk5 : PermuteDimensions
  cfblk6 : Sum  Inputs=+-
  cfblk7 : Sum  Inputs=+-
  cfblk8 : Sum  Inputs=+-
  cfblk9 : Gain  Gain=[720037740.520743]
  cfblk2 : Outport
  wires:
  cfblk9/1 -> cfblk8/1
  cfblk10/1 -> cfblk2/1
  cfblk4/1 -> cfblk3/1
  cfblk1/1 -> cfblk7/1, cfblk6/2
  cfblk8/1 -> cfblk4/1
  cfblk5/1 -> cfblk9/1
  cfblk11/1 -> cfblk7/2
  cfblk7/1 -> cfblk5/1
  cfblk3/1 -> cfblk6/1
  cfblk6/1 -> cfblk12/1
  cfblk12/1 -> cfblk8/2

== system Sample594/cfblk7/cfblk13/cfblk12/cfblk12 ==
  cfblk1 : Inport
  cfblk7 : Inport  Port=2
  cfblk3 : simulink/Math Operations/MinMax Running Resettable  Function=min  vinit=0.0
  cfblk4 : Signum
  cfblk5 : Bias  Bias=[-191921402.773867]
  cfblk6 : MinMax  Function=max  Inputs=3
  cfblk8 : Delay  SampleTime=1
  cfblk2 : Outport
  wires:
  cfblk3/1 -> cfblk2/1
  cfblk1/1 -> cfblk6/1, cfblk6/2
  cfblk4/1 -> cfblk5/1, cfblk8/1
  cfblk5/1 -> cfblk3/1
  cfblk7/1 -> cfblk3/2
  cfblk6/1 -> cfblk4/1
  cfblk8/1 -> cfblk6/3

== system Sample594/cfblk7/cfblk13/cfblk12/cfblk16 ==
  cfblk1 : Inport
  cfblk14 : Inport  Port=2
  Action Port : ActionPort  ActionPortLabel=if(u1 >= 0)
  cfblk10 : ComplexToRealImag
  cfblk11 : Math  Operator=magnitude^2  SaturateOnIntegerOverflow=on
  cfblk12 : Product  Inputs=**
  cfblk13 : Constant  Value=[43659368.130920]  SampleTime=1
  cfblk17 : Delay
  cfblk3 : simulink/Discrete/Transfer Fcn Lead or Lag  PoleZ=0.95  ZeroZ=0.75  ICPrevOutput=0.0  ICPrevInput=0.0  DoSatur=off
      settings: SourceProductBaseCode=SL
  cfblk4 : Sqrt  Operator=rSqrt  AlgorithmType=Newton-Raphson  SaturateOnIntegerOverflow=on
  cfblk5 : Polyval  Coefs=[ +2.081618890e-019, -1.441693666e-014, +4.719686976e-010, -8.536869453e-006, +1.621573104e-001, -8.087801117e+001 ]
  cfblk6 : Sum  Inputs=|++
  cfblk7 : Product
  cfblk8 : Sqrt  Operator=rSqrt  AlgorithmType=Newton-Raphson  SaturateOnIntegerOverflow=on
  cfblk9 : Sin  TimeSource=Use external signal  SampleTime=0
  cfblk2 : Outport
  cfblk15 : Outport  Port=2
  cfblk16 : Outport  Port=3
  wires:
  cfblk11/1 -> cfblk3/1
  cfblk13/1 -> cfblk15/1, cfblk6/2
  cfblk14/1 -> cfblk8/1
  cfblk7/1 -> cfblk12/1
  cfblk9/1 -> cfblk11/1, cfblk16/1
  cfblk1/1 -> cfblk7/1
  cfblk8/1 -> cfblk10/1
  cfblk3/1 -> cfblk6/1
  cfblk4/1 -> cfblk9/1
  cfblk6/1 -> cfblk7/2
  cfblk12/1 -> cfblk5/1
  cfblk10/1 -> cfblk2/1
  cfblk10/2 -> cfblk4/1
  cfblk5/1 -> cfblk17/1
  cfblk17/1 -> cfblk12/2

== system Sample594/cfblk7/cfblk13/cfblk12/cfblk17 ==
  cfblk1 : Inport
  cfblk8 : Inport  Port=2
  Action Port : ActionPort  ActionPortLabel=else
  cfblk3 : simulink/Discrete/Difference  ICPrevInput=0.0  OutMin=[]  OutMax=[]  OutDataTypeStr=Inherit: Inherit via back propagation  OutDataType=fixdt(1, 16)  OutScaling=2^-10  DoSatur=off
  cfblk4 : simulink/Discrete/Transfer Fcn Real Zero  ZeroZ=0.75  ICPrevInput=0.0  DoSatur=off
      settings: SourceProductBaseCode=SL
  cfblk5 : Sqrt  Operator=rSqrt  AlgorithmType=Newton-Raphson  SaturateOnIntegerOverflow=on
  cfblk6 : Sqrt  SaturateOnIntegerOverflow=on
  cfblk7 : Constant  Value=[-523203136.993245]  SampleTime=1
  cfblk2 : Outport
  cfblk9 : Outport  Port=2
  wires:
  cfblk8/1 -> cfblk6/1
  cfblk3/1 -> cfblk2/1
  cfblk4/1 -> cfblk3/1
  cfblk1/1 -> cfblk4/1
  cfblk6/1 -> cfblk5/1
  cfblk5/1 -> cfblk9/1

== system Sample594/cfblk7/cfblk13/cfblk12/cfblk7 ==
  cfblk1 : Inport
  cfblk9 : Inport  Port=2
  cfblk3 : DiscreteFir  SampleTime=1
  cfblk4 : Bias  Bias=[548395850.268470]
  cfblk5 : Reshape
  cfblk6 : Product
  cfblk7 : Polyval  Coefs=[ +2.081618890e-019, -1.441693666e-014, +4.719686976e-010, -8.536869453e-006, +1.621573104e-001, -8.087801117e+001 ]
  cfblk8 : Constant  Value=[-638304028.117423]  SampleTime=1
  cfblk2 : Outport
  cfblk10 : Outport  Port=2
  cfblk11 : Outport  Port=3
  wires:
  cfblk9/1 -> cfblk6/1
  cfblk1/1 -> cfblk7/1
  cfblk5/1 -> cfblk11/1
  cfblk7/1 -> cfblk6/2
  cfblk6/1 -> cfblk4/1
  cfblk3/1 -> cfblk5/1
  cfblk4/1 -> cfblk10/1, cfblk2/1
  cfblk8/1 -> cfblk3/1

== system Sample594/cfblk7/cfblk13/cfblk12/cfblk8 ==
  cfblk1 : Inport
  cfblk10 : Inport  Port=2
  cfblk11 : Inport  Port=3
  cfblk12 : Inport  Port=4
  cfblk13 : Inport  Port=5
  cfblk14 : Inport  Port=6
  cfblk15 : Inport  Port=7
  cfblk3 : DiscreteZeroPole  Poles=[0 0.5]  Gain=1
  cfblk4 : DiscreteZeroPole  Poles=[0 0.5]  Gain=1
  cfblk5 : pid_lib/PID Controller  Controller=PID  Form=Parallel  TimeDomain=Discrete-time  UseExternalTs=off  SampleTime=1  IntegratorMethod=Forward Euler  FilterMethod=Forward Euler  ControllerParametersSource=internal  P=1  I=1  D=0  UseFilter=on  N=100  TunerSelectOption=Transfer Function Based (PID Tuner App)  InitialConditionSource=internal  InitialConditionForIntegrator=0  InitialConditionForFilter=0  DifferentiatorICPrevScaledInput=0  ExternalReset=none  TrackingMode=off  Kt=1  LimitOutput=off  SatLimitsSource=internal  UpperSaturationLimit=inf  LowerSaturationLimit=-inf  LinearizeAsGain=off  AntiWindupMode=none  Kb=1  POutMin=[]  POutMax=[]  IOutMin=[]  IOutMax=[]  DOutMin=[]  DOutMax=[]  NOutMin=[]  NOutMax=[]  SumOutMin=[]  SumOutMax=[]  SaturationOutMin=[]  SaturationOutMax=[]  PParamMin=[]  PParamMax=[]  IParamMin=[]  IParamMax=[]  DParamMin=[]  DParamMax=[]  NParamMin=[]  NParamMax=[]  KbParamMin=[]  KbParamMax=[]  KtParamMin=[]  KtParamMax=[]  KbOutMin=[]  KbOutMax=[]  KtOutMin=[]  KtOutMax=[]  IntegratorOutMin=[]  IntegratorOutMax=[]  FilterOutMin=[]  FilterOutMax=[]  SumI1OutMin=[]  SumI1OutMax=[]  SumI2OutMin=[]  SumI2OutMax=[]  SumI3OutMin=[]  SumI3OutMax=[]  SumI4OutMin=[]  SumI4OutMax=[]  SumDOutMin=[]  SumDOutMax=[]  DifferentiatorOutMin=[]  DifferentiatorOutMax=[]  FilterDiffOutCoefMin=[]  FilterDiffOutCoefMax=[]  ReciprocalOutMin=[]  ReciprocalOutMax=[]  SumDenOutMin=[]  SumDenOutMax=[]  SumNumOutMin=[]  SumNumOutMax=[]  DivideOutMin=[]  DivideOutMax=[]  UdiffTsProdOutMin=[]  UdiffTsProdOutMax=[]  NTsProdOutMin=[]  NTsProdOutMax=[]  UintegralTsProdOutMin=[]  UintegralTsProdOutMax=[]  UngainTsProdOutMin=[]  UngainTsProdOutMax=[]  IntegratorContinuousStateAttributes=''  IntegratorStateMustResolveToSignalObject=off  IntegratorRTWStateStorageClass=Auto  FilterContinuousStateAttributes=''  FilterStateMustResolveToSignalObject=off  FilterRTWStateStorageClass=Auto  ParallelPVariant=InternalParameters  IdealPVariant=Disabled  IVariant=InternalParameters  DVariant=InternalParameters  IntegratorVariant=Discrete  SatVariant=Disabled  AWVariant=Passthrough  PCopyVariant=Disabled  TRVariant=Disabled  FdbkBlocksVariant=Forward  IdealPFdbkVariant=Disabled  SatFdbkVariant=Disabled  DerivativeFilterVariant=ForwardEulerFilter  NVariant=InternalParameters  NCopyVariant=Disabled  FilterICVariant=InternalICsFilter  IntegratorICVariant=InternalICs  ExternalResetVariant=Disabled  TRSumVariant=Passthrough  SumFdbkVariant=Disabled  SumVariant=Sum_PID  TsampFilterVariant=InternalTs  TsampNgainVariant=Passthrough  TsampIntegralVariant=Passthrough  ExternalSaturationOutDataTypeStr=Inherit: Same as second input
  cfblk6 : Polyval  Coefs=[ +2.081618890e-019, -1.441693666e-014, +4.719686976e-010, -8.536869453e-006, +1.621573104e-001, -8.087801117e+001 ]
  cfblk7 : Bias  Bias=[-408530010.181376]
  cfblk8 : Bias  Bias=[476700600.959226]
  cfblk9 : Constant  Value=[-815016053.231957]  SampleTime=1
  cfblk2 : Outport
  wires:
  cfblk6/1 -> cfblk2/1
  cfblk14/1 -> cfblk6/1
  cfblk8/1 -> cfblk5/1
  cfblk1/1 -> cfblk3/1
  cfblk3/1 -> cfblk4/1
  cfblk4/1 -> cfblk8/1
  cfblk15/1 -> cfblk7/1

== system Sample594/cfblk7/cfblk13/cfblk12/cfblk9 ==
  cfblk1 : Inport
  cfblk6 : Inport  Port=2
  cfblk7 : Inport  Port=3
  cfblk3 : Sqrt  SaturateOnIntegerOverflow=on
  cfblk4 : Sin  TimeSource=Use external signal  SampleTime=0
  cfblk5 : Gain  Gain=[134197400.326504]
  cfblk2 : Outport
  cfblk8 : Outport  Port=2
  wires:
  cfblk6/1 -> cfblk8/1
  cfblk7/1 -> cfblk5/1
  cfblk5/1 -> cfblk3/1
  cfblk4/1 -> cfblk2/1
  cfblk1/1 -> cfblk4/1

== system Sample594/cfblk7/cfblk13/cfblk17/cfblk10 ==
  cfblk1 : Inport
  cfblk7 : Inport  Port=2
  cfblk3 : simulink/Discrete/Transfer Fcn Real Zero  ZeroZ=0.75  ICPrevInput=0.0  DoSatur=off
      settings: SourceProductBaseCode=SL
  cfblk4 : Squeeze
  cfblk5 : Sqrt  SaturateOnIntegerOverflow=on
  cfblk6 : Constant  Value=[234560851.981873]  SampleTime=1
  cfblk2 : Outport
  wires:
  cfblk7/1 -> cfblk4/1
  cfblk3/1 -> cfblk2/1
  cfblk5/1 -> cfblk3/1
  cfblk4/1 -> cfblk5/1

== system Sample594/cfblk7/cfblk13/cfblk17/cfblk11 ==
  cfblk1 : Inport
  cfblk12 : Inport  Port=2
  cfblk13 : Inport  Port=3
  cfblk10 : Constant  Value=[501293799.661589]  SampleTime=1
  cfblk11 : Constant  Value=[47160282.083164]  SampleTime=1
  cfblk3 : DiscreteStateSpace  SampleTime=-1
  cfblk4 : pid_lib/PID Controller (2DOF)  Controller=PID  Form=Parallel  TimeDomain=Discrete-time  UseExternalTs=off  SampleTime=-1  IntegratorMethod=Forward Euler  FilterMethod=Forward Euler  ControllerParametersSource=internal  P=1  I=1  D=0  UseFilter=on  N=100  b=1  c=1  TunerSelectOption=Transfer Function Based (PID Tuner App)  InitialConditionSource=internal  InitialConditionForIntegrator=0  InitialConditionForFilter=0  DifferentiatorICPrevScaledInput=0  ExternalReset=none  TrackingMode=off  Kt=1  LimitOutput=off  SatLimitsSource=internal  UpperSaturationLimit=inf  LowerSaturationLimit=-inf  LinearizeAsGain=off  AntiWindupMode=none  Kb=1  POutMin=[]  POutMax=[]  IOutMin=[]  IOutMax=[]  DOutMin=[]  DOutMax=[]  NOutMin=[]  NOutMax=[]  bOutMin=[]  bOutMax=[]  cOutMin=[]  cOutMax=[]  SumOutMin=[]  SumOutMax=[]  SaturationOutMin=[]  SaturationOutMax=[]  PParamMin=[]  PParamMax=[]  IParamMin=[]  IParamMax=[]  DParamMin=[]  DParamMax=[]  NParamMin=[]  NParamMax=[]  bParamMin=[]  bParamMax=[]  cParamMin=[]  cParamMax=[]  KbParamMin=[]  KbParamMax=[]  KtParamMin=[]  KtParamMax=[]  KbOutMin=[]  KbOutMax=[]  KtOutMin=[]  KtOutMax=[]  IntegratorOutMin=[]  IntegratorOutMax=[]  FilterOutMin=[]  FilterOutMax=[]  SumI1OutMin=[]  SumI1OutMax=[]  SumI2OutMin=[]  SumI2OutMax=[]  SumI3OutMin=[]  SumI3OutMax=[]  SumI4OutMin=[]  SumI4OutMax=[]  SumDOutMin=[]  SumDOutMax=[]  Sum1OutMin=[]  Sum1OutMax=[]  Sum2OutMin=[]  Sum2OutMax=[]  Sum3OutMin=[]  Sum3OutMax=[]  DifferentiatorOutMin=[]  DifferentiatorOutMax=[]  FilterDiffOutCoefMin=[]  FilterDiffOutCoefMax=[]  ReciprocalOutMin=[]  ReciprocalOutMax=[]  SumDenOutMin=[]  SumDenOutMax=[]  SumNumOutMin=[]  SumNumOutMax=[]  DivideOutMin=[]  DivideOutMax=[]  UdiffTsProdOutMin=[]  UdiffTsProdOutMax=[]  NTsProdOutMin=[]  NTsProdOutMax=[]  UintegralTsProdOutMin=[]  UintegralTsProdOutMax=[]  UngainTsProdOutMin=[]  UngainTsProdOutMax=[]  IntegratorContinuousStateAttributes=''  IntegratorStateMustResolveToSignalObject=off  IntegratorRTWStateStorageClass=Auto  FilterContinuousStateAttributes=''  FilterStateMustResolveToSignalObject=off  FilterRTWStateStorageClass=Auto  ParallelPVariant=InternalParameters  IdealPVariant=Disabled  IVariant=InternalParameters  DVariant=InternalParameters  bVariant=InternalParameters  cVariant=InternalParameters  IntegratorVariant=Discrete  SatVariant=Disabled  AWVariant=Passthrough  PCopyVariant=Disabled  TRVariant=Disabled  FdbkBlocksVariant=Forward  IdealPFdbkVariant=Disabled  SatFdbkVariant=Disabled  DerivativeFilterVariant=ForwardEulerFilter  NVariant=InternalParameters  NCopyVariant=Disabled  FilterICVariant=InternalICsFilter  IntegratorICVariant=InternalICs  ExternalResetVariant=Disabled  TRSumVariant=Passthrough  SumFdbkVariant=Disabled  SumVariant=Sum_PID  TsampFilterVariant=InternalTs  TsampNgainVariant=Passthrough  TsampIntegralVariant=Passthrough  ExternalSaturationOutDataTypeStr=Inherit: Same as second input
      settings: SourceProductBaseCode=SL
  cfblk5 : UnitDelay  SampleTime=-1  HasFrameUpgradeWarning=on
  cfblk6 : MinMax  Inputs=2
  cfblk7 : UnaryMinus
  cfblk8 : PermuteDimensions
  cfblk9 : Squeeze
  cfblk2 : Outport
  wires:
  cfblk5/1 -> cfblk6/1
  cfblk1/1 -> cfblk6/2
  cfblk13/1 -> cfblk2/1
  cfblk6/1 -> cfblk8/1
  cfblk12/1 -> cfblk4/1
  cfblk9/1 -> cfblk3/1
  cfblk8/1 -> cfblk4/2
  cfblk7/1 -> cfblk9/1
  cfblk11/1 -> cfblk5/1
  cfblk10/1 -> cfblk7/1

== system Sample594/cfblk7/cfblk13/cfblk17/cfblk12 ==
  cfblk1 : Inport
  cfblk15 : Inport  Port=2
  cfblk16 : Inport  Port=3
  cfblk10 : Gain  Gain=[-705607098.203998]
  cfblk11 : Constant  Value=[503433820.870529]  SampleTime=1
  cfblk12 : Constant  Value=[-960687358.772930]  SampleTime=1
  cfblk13 : Constant  Value=[693349242.694060]  SampleTime=1
  cfblk14 : Constant  Value=[423185679.840892]  SampleTime=1
  cfblk3 : DiscreteFir
  cfblk4 : Math  Operator=log10  SaturateOnIntegerOverflow=on
  cfblk5 : Polyval  Coefs=[ +2.081618890e-019, -1.441693666e-014, +4.719686976e-010, -8.536869453e-006, +1.621573104e-001, -8.087801117e+001 ]
  cfblk6 : Product  Inputs=*
  cfblk7 : Sqrt  Operator=rSqrt  AlgorithmType=Newton-Raphson  SaturateOnIntegerOverflow=on
  cfblk8 : Sin  TimeSource=Use external signal  SampleTime=0
  cfblk9 : Abs
  cfblk2 : Outport
  wires:
  cfblk16/1 -> cfblk4/1
  cfblk4/1 -> cfblk5/1
  cfblk9/1 -> cfblk2/1
  cfblk3/1 -> cfblk10/1
  cfblk10/1 -> cfblk8/1
  cfblk11/1 -> cfblk6/1
  cfblk7/1 -> cfblk9/1
  cfblk12/1 -> cfblk3/1
  cfblk15/1 -> cfblk7/1

== system Sample594/cfblk7/cfblk13/cfblk17/cfblk13 ==
  cfblk1 : Inport
  cfblk6 : Inport  Port=2
  cfblk7 : Inport  Port=3
  cfblk3 : Polyval  Coefs=[ +2.081618890e-019, -1.441693666e-014, +4.719686976e-010, -8.536869453e-006, +1.621573104e-001, -8.087801117e+001 ]
  cfblk4 : DotProduct  InputSameDT=on  OutDataTypeStr=Inherit: Inherit via internal rule
  cfblk5 : Sum  Inputs=--
  cfblk2 : Outport
  wires:
  cfblk3/1 -> cfblk4/1
  cfblk7/1 -> cfblk2/1, cfblk5/2
  cfblk6/1 -> cfblk4/2
  cfblk4/1 -> cfblk5/1
  cfblk1/1 -> cfblk3/1

== system Sample594/cfblk7/cfblk13/cfblk17/cfblk9 ==
  cfblk1 : Inport
  cfblk3 : Delay
  cfblk4 : Delay  DelayLengthSource=Input port
      settings: InputPortMap=u0,p1
  cfblk5 : Sin  TimeSource=Use external signal  SampleTime=0
  cfblk6 : Gain  Gain=[-61022936.009616]
  cfblk7 : simulink/Math Operations/Slider Gain  gain=1  low=0  high=2
  cfblk8 : Constant  Value=[879417360.853315]  SampleTime=1
  cfblk2 : Outport
  cfblk9 : Outport  Port=2
  cfblk10 : Outport  Port=3
  wires:
  cfblk3/1 -> cfblk5/1
  cfblk7/1 -> cfblk2/1, cfblk4/2
  cfblk8/1 -> cfblk9/1
  cfblk1/1 -> cfblk6/1
  cfblk5/1 -> cfblk4/1, cfblk7/1
  cfblk4/1 -> cfblk10/1
  cfblk6/1 -> cfblk3/1

== system Sample594/cfblk7/cfblk13/cfblk18/cfblk5 ==
  cfblk1 : Inport
  cfblk8 : Inport  Port=2
  cfblk9 : Inport  Port=3
  cfblk10 : Inport  Port=4
  cfblk3 : Squeeze
  cfblk4 : ComplexToRealImag
  cfblk5 : Trigonometry
  cfblk6 : Constant  Value=[92057409.995910]  SampleTime=1
  cfblk7 : Constant  Value=[-354168129.248079]  SampleTime=1
  cfblk2 : Outport
  cfblk11 : Outport  Port=2
  wires:
  cfblk9/1 -> cfblk2/1
  cfblk5/1 -> cfblk3/1
  cfblk6/1 -> cfblk4/1
  cfblk1/1 -> cfblk5/1
  cfblk3/1 -> cfblk11/1

== system Sample594/cfblk7/cfblk13/cfblk18/cfblk6 ==
  cfblk1 : Inport
  cfblk5 : Inport  Port=2
  cfblk6 : Inport  Port=3
  cfblk3 : Sum  Inputs=|++
  cfblk4 : Trigonometry
  cfblk2 : Outport
  cfblk7 : Outport  Port=2
  wires:
  cfblk6/1 -> cfblk7/1
  cfblk1/1 -> cfblk3/1
  cfblk5/1 -> cfblk4/1
  cfblk4/1 -> cfblk3/2
  cfblk3/1 -> cfblk2/1

== system Sample594/cfblk7/cfblk13/cfblk18/cfblk7 ==
  cfblk1 : Inport
  cfblk7 : Inport  Port=2
  cfblk8 : Inport  Port=3
  cfblk9 : Inport  Port=4
  cfblk3 : simulink/Discrete/Transfer Fcn First Order  PoleZ=0.95  ICPrevOutput=0.0  DoSatur=off
  cfblk4 : Delay
  cfblk5 : ComplexToMagnitudeAngle
  cfblk6 : Constant  Value=[-513590252.558153]  SampleTime=1
  cfblk2 : Outport
  wires:
  cfblk7/1 -> cfblk3/1
  cfblk8/1 -> cfblk2/1
  cfblk3/1 -> cfblk4/1
  cfblk9/1 -> cfblk5/1

== system Sample594/cfblk7/cfblk13/cfblk18/cfblk8 ==
  cfblk1 : Inport
  cfblk9 : Inport  Port=2
  cfblk3 : DiscreteIntegrator  SampleTime=-1  ICPrevOutput=DiscIntNeverNeededParam  ICPrevScaledInput=DiscIntNeverNeededParam
  cfblk4 : simulink/Math Operations/Slider Gain  gain=1  low=0  high=2
  cfblk5 : Squeeze
  cfblk6 : DotProduct  InputSameDT=on  OutDataTypeStr=Inherit: Inherit via internal rule
  cfblk7 : Sin  TimeSource=Use external signal  SampleTime=0
  cfblk8 : Math  Operator=square  SaturateOnIntegerOverflow=on
  cfblk2 : Outport
  wires:
  cfblk1/1 -> cfblk7/1
  cfblk4/1 -> cfblk6/1
  cfblk6/1 -> cfblk2/1
  cfblk8/1 -> cfblk3/1
  cfblk3/1 -> cfblk6/2
  cfblk9/1 -> cfblk5/1
  cfblk5/1 -> cfblk4/1
  cfblk7/1 -> cfblk8/1
